simulink model "RGB_UART"  (R2020b)
settings: Solver=VariableStepAuto  StartTime=0.0  StopTime=inf  RelTol=1e-3
undefined symbols (not defined in the file): serial
libraries: instrumentlib x2
settings Model: Creator=ashle  LastModifiedBy=adria
settings SFSimCC: CustomCodeUndefinedFunction=UseInterfaceOnly

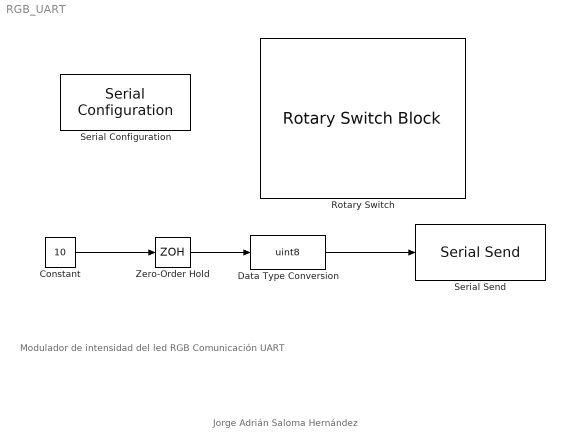
== system RGB_UART ==
  note: Jorge Adrián Saloma Hernández
  note: Modulador de intensidad del led RGB
      | Comunicación UART
  "Constant " : Constant  Value=10
  Data Type Conversion : DataTypeConversion  OutDataTypeStr=uint8
  Rotary Switch : RotarySwitchBlock
      settings: Values={{'0 %', '10 %', '20 %', '30 %', '40 %', '50 %', '60 %', '70 %', '80 %', '90 %', '100 %', 'Rojo', 'Verde', 'Azul'}, [1 10 20 30 40 50 60 70 80 90 100 114 103 98]}
  "Serial Configuration " : instrumentlib/Serial Configuration  Priority=-200000  ComPortMenu=<Please select a port...>  ComPort=COM10  ObjConstructor=serial('COM10');  BaudRate=9600  DataBits=8  Parity=none  StopBits=1  FlowControl=none  Timeout=10  ByteOrder=LittleEndian
  "Serial Send " : instrumentlib/Serial Send  ComPortMenu=<Please select a port...>  ComPort=COM10  ObjConstructor=serial('COM10');  Terminator=<none>  EnableBlockingMode=on
  "Zero-Order Hold " : ZeroOrderHold  SampleTime=0.5
  wires:
  "Constant "/1 -> "Zero-Order Hold "/1
  "Zero-Order Hold "/1 -> Data Type Conversion/1
  Data Type Conversion/1 -> "Serial Send "/1
